simulink model "ModuladorProyectoFinal"  (R2021a)
settings: Solver=VariableStepAuto  StartTime=0.0  StopTime=3  RelTol=1e-3
libraries: commutil2 x3, commdigbbndpm3 x1, dspvision x1
settings Model: Creator=daddy  LastModifiedBy=daddy

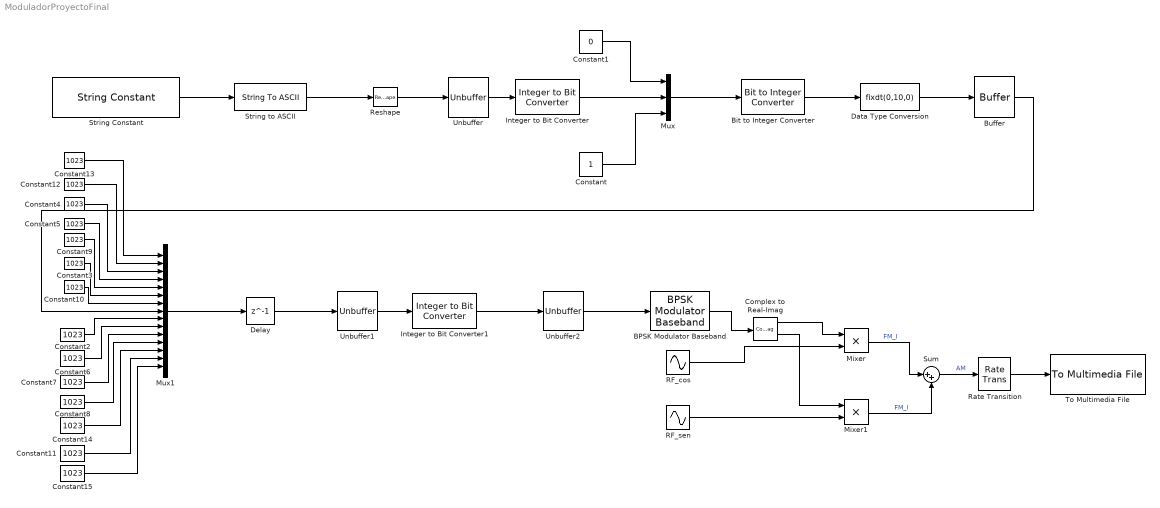
== system ModuladorProyectoFinal ==
  "\tMixer" : Product
  "\tMixer1" : Product
  BPSK Modulator Baseband : commdigbbndpm3/BPSK Modulator Baseband  Ph=0  outDtype=Fixed-point  outWordLen=8  outUDDataType=sfix(16)  outFracLenMode=User-defined  outFracLen=0  outDataTypeStr=fixdt(1,8,0)  outLastDataTypeStr=fixdt(1,8,0)
  Bit to Integer Converter : commutil2/Bit to Integer Converter  nbits=10  bitOrder=MSB first  signedOutputValues=Unsigned  outDtype=Inherit via internal rule  outDtypeSigned=Inherit via internal rule
  Buffer : Buffer  N=4  OutputFrames=off
  Complex to Real-Imag : ComplexToRealImag
  Constant : Constant  OutDataTypeStr=boolean
  Constant1 : Constant  Value=0  OutDataTypeStr=boolean
  Constant{2..15} (14 alike) : Constant  Value=1023  OutDataTypeStr=fixdt(0,10)
  Data Type Conversion : DataTypeConversion  OutDataTypeStr=fixdt(0,10,0)
  Delay : Delay  DelayLength=1  SampleTime=1
  Integer to Bit Converter : commutil2/Integer to Bit Converter  nbits=8  signedInputValues=Unsigned  bitOrder=MSB first  outDtype=boolean
  Integer to Bit Converter1 : commutil2/Integer to Bit Converter  nbits=10  signedInputValues=Unsigned  bitOrder=MSB first  outDtype=boolean
  Mux : Mux  Inputs=3
  Mux1 : Mux  Inputs=15
  RF_cos : Sin  Frequency=2*pi*4500  Phase=pi/2  SampleTime=0
  RF_sen : Sin  Amplitude=-1  Frequency=2*pi*4500  SampleTime=0
  Rate Transition : RateTransition  OutPortSampleTime=1/44100
  Reshape : Reshape
  String Constant : StringConstant  String='Hola'
  String to ASCII : StringToASCII  OutputVectorSize=4
  Sum : Sum  Inputs=|++
  To Multimedia File : dspvision/To Multimedia File  outputFilename=C:\Users\daddy\Downloads\ProyectoSC\audio.wav  streamSelection=Audio only  videoCompressor=None (uncompressed)  audioCompressor=None (uncompressed)  imagePorts=Separate color signals  fileType=WAV  audioDatatype=16-bit integer  fourcc=RGB  videoQuality=75  mj2000CompFactor=10
  Unbuffer : Unbuffer
  Unbuffer1 : Unbuffer
  Unbuffer2 : Unbuffer
  wires:
  Mux1/1 -> Delay/1
  Unbuffer1/1 -> Integer to Bit Converter1/1
  Delay/1 -> Unbuffer1/1
  Constant1/1 -> Mux/1
  Integer to Bit Converter1/1 -> Unbuffer2/1
  BPSK Modulator Baseband/1 -> Complex to Real-Imag/1
  RF_sen/1 -> "\tMixer1"/2
  "\tMixer1"/1 -> Sum/2  "FM_I"
  Complex to Real-Imag/2 -> "\tMixer1"/1
  "\tMixer"/1 -> Sum/1  "FM_I"
  RF_cos/1 -> "\tMixer"/2
  Data Type Conversion/1 -> Buffer/1
  Reshape/1 -> Unbuffer/1
  Mux/1 -> Bit to Integer Converter/1
  Unbuffer2/1 -> BPSK Modulator Baseband/1
  Buffer/1 -> Mux1/8
  Constant/1 -> Mux/3
  Complex to Real-Imag/1 -> "\tMixer"/1
  Bit to Integer Converter/1 -> Data Type Conversion/1
  String to ASCII/1 -> Reshape/1
  Unbuffer/1 -> Integer to Bit Converter/1
  String Constant/1 -> String to ASCII/1
  Integer to Bit Converter/1 -> Mux/2
  Sum/1 -> Rate Transition/1  "AM"
  Rate Transition/1 -> To Multimedia File/1
  Constant13/1 -> Mux1/1
  Constant12/1 -> Mux1/2
  Constant5/1 -> Mux1/4
  Constant3/1 -> Mux1/6
  Constant2/1 -> Mux1/9
  Constant6/1 -> Mux1/10
  Constant7/1 -> Mux1/11
  Constant8/1 -> Mux1/12
  Constant14/1 -> Mux1/13
  Constant11/1 -> Mux1/14
  Constant15/1 -> Mux1/15
  Constant4/1 -> Mux1/3
  Constant9/1 -> Mux1/5
  Constant10/1 -> Mux1/7
